simulink model "lab3_simulink"  (R2015a)
settings: Solver=ode45  StartTime=0.0  StopTime=inf  RelTol=1e-3
undefined symbols (not defined in the file or in its folder): currentCFG_lab3_simulink_UB, fdesignblkfcn, gcbh, UB
libraries: dspstat3 x2, gtecHighspeedLib x1, gUSBamplib x1
settings Model: Creator=circuit  LastModifiedBy=circuit

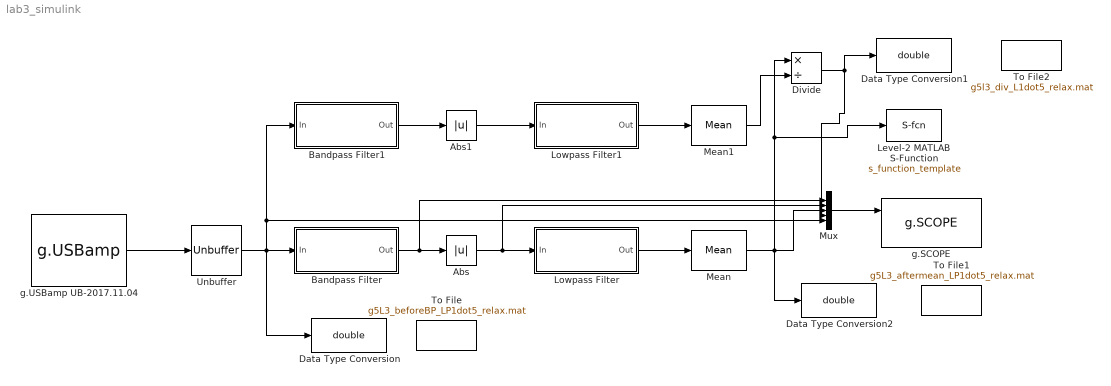
== system lab3_simulink ==
  Abs : Abs
  Abs1 : Abs
  Bandpass Filter : Subsystem  DialogController=fdesignblkfcn  InitFcn=fdesignblkfcn(gcbh, {'InitFcn'});  mask(Bandpass Filter){}
      mask help: Design a bandpass filter
      settings: CopyFcn=fdesignblkfcn(gcbh, {'CopyFcn'});
      mask Help: helpview(mapfilelocation('dsp'), 'dspbandpassfilter');
      mask Display: disp('Bandpass');
  Bandpass Filter1 : Subsystem  DialogController=fdesignblkfcn  InitFcn=fdesignblkfcn(gcbh, {'InitFcn'});  mask(Bandpass Filter){}
      mask help: Design a bandpass filter
      settings: CopyFcn=fdesignblkfcn(gcbh, {'CopyFcn'});
      mask Help: helpview(mapfilelocation('dsp'), 'dspbandpassfilter');
      mask Display: disp('Bandpass');
  Data Type Conversion : DataTypeConversion  OutDataTypeStr=double
  Data Type Conversion1 : DataTypeConversion  OutDataTypeStr=double
  Data Type Conversion2 : DataTypeConversion  OutDataTypeStr=double
  Divide : Product  Inputs=*/
  Level-2 MATLAB S-Function : M-S-Function  FunctionName=s_function_template
  Lowpass Filter : Subsystem  DialogController=fdesignblkfcn  InitFcn=fdesignblkfcn(gcbh, {'InitFcn'});  mask(Lowpass Filter){}
      mask help: Design a lowpass filter
      settings: CopyFcn=fdesignblkfcn(gcbh, {'CopyFcn'});
      mask Help: helpview(mapfilelocation('dsp'), 'dsplowpassfilter');
      mask Display: disp('Lowpass')
  Lowpass Filter1 : Subsystem  DialogController=fdesignblkfcn  InitFcn=fdesignblkfcn(gcbh, {'InitFcn'});  mask(Lowpass Filter){}
      mask help: Design a lowpass filter
      settings: CopyFcn=fdesignblkfcn(gcbh, {'CopyFcn'});
      mask Help: helpview(mapfilelocation('dsp'), 'dsplowpassfilter');
      mask Display: disp('Lowpass')
  Mean : dspstat3/Mean  run=off  reset_popup=None  InputProcessing=Columns as channels (frame based)  directionMode=Each row  dimension=1  treatSBRowAsCol=off  roiEnable=off  roiType=Rectangles  roiPortion=Entire ROI  roiOutput=Individual statistics for each ROI  roiFlag=off  outputDataTypeStr=Inherit: Same as accumulator  outputLastDataTypeStr=Inherit: Same as accumulator  outputMin=[]  outputMax=[]  roundingMode=Floor  overflowMode=off
  Mean1 : dspstat3/Mean  run=off  reset_popup=None  InputProcessing=Columns as channels (frame based)  directionMode=Each row  dimension=1  treatSBRowAsCol=off  roiEnable=off  roiType=Rectangles  roiPortion=Entire ROI  roiOutput=Individual statistics for each ROI  roiFlag=off  outputDataTypeStr=Inherit: Same as accumulator  outputLastDataTypeStr=Inherit: Same as accumulator  outputMin=[]  outputMax=[]  roundingMode=Floor  overflowMode=off
  Mux : Mux  Inputs=5
  To File : ToFile  Filename=g5L3_beforeBP_LP1dot5_relax.mat
  To File1 : ToFile  Filename=g5L3_aftermean_LP1dot5_relax.mat
  To File2 : ToFile  Filename=g5l3_div_L1dot5_relax.mat
  Unbuffer : Unbuffer  SampleBasedProcessing=Same as frame based
  g.SCOPE : gtecHighspeedLib/g.SCOPE
  g.USBamp UB-2017.11.04 : gUSBamplib/g.USBamp  cfg=currentCFG_lab3_simulink_UB-2017.11.04.cfg  snr=UB-2017.11.04
  wires:
  g.USBamp UB-2017.11.04/1 -> Unbuffer/1
  Unbuffer/1 -> Mux/5, Bandpass Filter1/1(In), Data Type Conversion/1, Bandpass Filter/1(In)
  Bandpass Filter/1(Out) -> Mux/1, Abs/1
  Abs/1 -> Mux/2, Lowpass Filter/1(In)
  Lowpass Filter/1(Out) -> Mean/1
  Mean/1 -> Data Type Conversion2/1, Level-2 MATLAB S-Function/1, Divide/1, Mux/3
  Mux/1 -> g.SCOPE/1
  Bandpass Filter1/1(Out) -> Abs1/1
  Abs1/1 -> Lowpass Filter1/1(In)
  Lowpass Filter1/1(Out) -> Mean1/1
  Mean1/1 -> Divide/2
  Divide/1 -> Mux/4, Data Type Conversion1/1

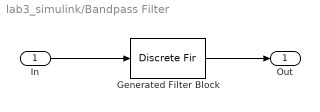
== system lab3_simulink/Bandpass Filter ==
  In : Inport
  Generated Filter Block : DiscreteFir  Tag=BlockMethodSubSystem  Coefficients=[-9.7066588284270048e-20 -1.9044423256952615e-05 -3.5042718823172766e-05 -4.4807719825143353e-05 -4.5567280109715214e-05 -3.5219071376037001e-05 -1.2566832640538831e-05 2.2477748850210183e-05 6.8746329856826839e-05 0.00012373897417179035 0.00018364330584267209 0.00024346501349722092 0.00029728073065491296 0.00033861492674996772 0.00036093040336402629 0.00035820828397517676 0.00032557941097418372 0.0002599565024307643 0.00016060705750857635 2.9602505805759997e-05 -0.00012791919221331879 -0.0003037315778843503 -0.00048677665569194672 -0.00066371693142762433 -0.00081977170567080506 -0.00093979727898122259 -0.001009541477783594 -0.0010169770659436866 -0.0009535992818404458 -0.00081556269315769165 -0.00060453385821604357 -0.0003281500071823974 1.3026996240236752e-18 0.00036091922099598179 0.00073127225101849466 0.0010849327740993554 0.0013949112623725371 0.0016355204203750049 0.0017846012484941276 0.0018256120596552639 0.0017493796388294641 0.001555327713823481 0.0012520329610216285 0.0008570109488230908 0.0003956999203308493 -0.00010031627534579806 -0.00059573006989686742 -0.0010543920094732372 -0.0014424118496333066 -0.0017312017957872362 -0.0019001726269555566 -0.0019388084332589079 -0.0018478882200996666 -0.0016396904076892227 -0.001337104385200843 -0.00097167455182888224 -0.00058070771915937872 -0.00020367438747929246 0.00012178182357201864 0.00036385360046769139 0.0005001989403861936 0.00052080130177256526 0.00042972187623116194 0.00024549074262117919 -6.5519947091882275e-19 -0.0002641002738728534 -0.00049735500687277676 -0.00064851427405487275 -0.00067018306520218889 -0.00052459840768443052 -0.0001889689641773141 0.00034019037963081895 0.0010442453309613309 0.001881563110656567 0.0027888299531657881 0.0036846416750790827 0.0044752368273439759 0.005062031623457793 0.0053504212256518489 0.0052591518963344946 0.0047294598397193298 0.0037331285176027498 0.0022786450626614109 0.00041474033817082845 -0.0017692281561480106 -0.0041463568556569328 -0.006558769024306554 -0.0088274099101692555 -0.010764498450602051 -0.012187803187946064 -0.012935697127694851 -0.012881808406232986 -0.011948036879107893 -0.010114760172307535 -0.0074272073597878765 -0.0039972267037172481 5.2492950851645509e-18 0.0043343631135675798 0.0087340107907784674 0.012902574048254914 0.016539329842932604 0.019360910578682729 0.021122975864728812 0.021640187116165964 0.020802878702137963 0.018589001722594856 0.015070218552972236 0.01041142840998025 0.0048634779709632522 -0.0012506785757137296 -0.0075555979048902606 -0.013647507136755674 -0.019121382890505238 -0.023599056579892485 -0.026756318585830479 -0.02834701119854131 -0.028222271249457628 -0.026343398434246216 -0.02278726318863793 -0.017743697271463996 -0.011504891841311345 -0.0044474179341587091 0.0029919623316966384 0.010345051741279927 0.017143542281197032 0.022950697652655314 0.027391135842824384 0.030176573770733611 0.031125676488437466 0.030176573770733611 0.027391135842824384 0.022950697652655314 0.017143542281197032 0.010345051741279927 0.0029919623316966384 -0.0044474179341587091 -0.011504891841311345 -0.017743697271463996 -0.02278726318863793 -0.026343398434246216 -0.028222271249457628 -0.02834701119854131 -0.026756318585830479 -0.023599056579892485 -0.019121382890505238 -0.013647507136755674 -0.0075555979048902606 -0.0012506785757137296 0.0048634779709632522 0.01041142840998025 0.015070218552972236 0.018589001722594856 0.020802878702137963 0.021640187116165964 0.021122975864728812 0.019360910578682729 0.016539329842932604 0.012902574048254914 0.0087340107907784674 0.0043343631135675798 5.2492950851645509e-18 -0.0039972267037172481 -0.0074272073597878765 -0.010114760172307535 -0.011948036879107893 -0.012881808406232986 -0.012935697127694851 -0.012187803187946064 -0.010764498450602051 -0.0088274099101692555 -0.006558769024306554 -0.0041463568556569328 -0.0017692281561480106 0.00041474033817082845 0.0022786450626614109 0.0037331285176027498 0.0047294598397193298 0.0052591518963344946 ...(+1817 chars)]  InputProcessing=Columns as channels (frame based)
  Out : Outport
  wires:
  In/1 -> Generated Filter Block/1
  Generated Filter Block/1 -> Out/1

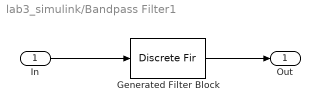
== system lab3_simulink/Bandpass Filter1 ==
  In : Inport
  Generated Filter Block : DiscreteFir  Tag=BlockMethodSubSystem  Coefficients=[-3.9043503106395059e-19 -7.5114923761997586e-05 -0.00012970926989761377 -0.00014606949442778406 -0.00011439896508069259 -3.5260344443637117e-05 8.0051557029435554e-05 0.00021140930249864958 0.000333790689790907 0.00042258113740490207 0.0004592101397287817 0.00043590560812563524 0.00035840430730046821 0.00024577958330473281 0.00012710940297959957 3.5414445181371547e-05 -4.995904333114398e-20 3.8863334376989846e-05 0.00015302162022515448 0.00032437590336606404 0.0005180515405703327 0.00068915525114254914 0.00079277447262141975 0.00079508692530240064 0.00068291437643216318 0.00046913655038040986 0.00019213465104790252 -9.1254063378733906e-05 -0.00031819201546482844 -0.00043512694543481635 -0.00041232096551297316 -0.0002538426644640838 3.5814836249778259e-18 0.00027919151213974422 0.00049876260278053136 0.00057884389263584697 0.00046544668648687939 0.00014675639116760108 -0.00033964304160326449 -0.00091132562644572401 -0.0014573282987569898 -0.0018631749037373697 -0.0020390866299198735 -0.00194452483268953 -0.0016025191355891963 -0.001099237431152839 -0.00056759386496819269 -0.00015763094535208865 0 -0.00017115615086961137 -0.00066918665182910024 -0.0014072608476174431 -0.0022278305628302426 -0.0029357410908228995 -0.0033435027143655905 -0.0033183670710667476 -0.0028195662306453326 -0.0019156126568000984 -0.00077575828959283732 0.00036427999882693573 0.0012557747791148068 0.0016977695616763443 0.0015905989231668213 0.00096826342113219891 -2.6354364596816659e-18 -0.0010416630459124207 -0.0018409403433254869 -0.0021141033846413331 -0.00168252853558822 -0.00052521318214320391 0.0012037448293721349 0.0031995824561332122 0.0050702251314133735 0.0064257287141921728 0.0069736219711172753 0.0065970709591041173 0.0053953855387002675 0.0036742149409364814 0.0018842658898869677 0.00051994874173862549 0 0.00055810037639090549 0.0021710251393396987 0.0045446075659693009 0.007165080986318643 0.0094079239968750117 0.010681746122149461 0.010574625825446118 0.0089674121418749399 0.0060840184071469412 0.0024619054376523448 -0.0011558936775474709 -0.0039867583877307607 -0.0053965252880086474 -0.0050657101633476698 -0.003092081836751504 4.2228921936307396e-18 0.0033528759939696652 0.0059570125198306449 0.0068839068792203315 0.0055187569845934793 0.0017372680468242762 -0.0040200979218537282 -0.010802545357728737 -0.017329928367361164 -0.022268336883116961 -0.024543667872978008 -0.023623130036761086 -0.019696280220295855 -0.013704582830915956 -0.0071987486173472988 -0.0020402937734144686 0 -0.002333132797226467 -0.0094228129569531496 -0.020575338090327674 -0.034025022595054896 -0.047165853317594202 -0.056980799081539031 -0.060596524457473204 -0.055860811648837987 -0.041829167575723386 -0.019058998402915254 0.010357175059788049 0.043039731361273592 0.07481739343065448 0.10138723110404568 0.11902229894830223 0.12519812101626032 0.11902229894830223 0.10138723110404568 0.07481739343065448 0.043039731361273592 0.010357175059788049 -0.019058998402915254 -0.041829167575723386 -0.055860811648837987 -0.060596524457473204 -0.056980799081539031 -0.047165853317594202 -0.034025022595054896 -0.020575338090327674 -0.0094228129569531496 -0.002333132797226467 0 -0.0020402937734144686 -0.0071987486173472988 -0.013704582830915956 -0.019696280220295855 -0.023623130036761086 -0.024543667872978008 -0.022268336883116961 -0.017329928367361164 -0.010802545357728737 -0.0040200979218537282 0.0017372680468242762 0.0055187569845934793 0.0068839068792203315 0.0059570125198306449 0.0033528759939696652 4.2228921936307396e-18 -0.003092081836751504 -0.0050657101633476698 -0.0053965252880086474 -0.0039867583877307607 -0.0011558936775474709 0.0024619054376523448 0.0060840184071469412 0.0089674121418749399 0.010574625825446118 0.010681746122149461 0.0094079239968750117 0.007165080986318643 0.0045446075659693009 0.0021710251393396987 0.00055810037639090549 0 0.00051994874173862549 0.0018842658898869677 0.0036742149409364814 0.0053953855387002675 0.0065970709591041173 ...(+1706 chars)]  InputProcessing=Columns as channels (frame based)
  Out : Outport
  wires:
  In/1 -> Generated Filter Block/1
  Generated Filter Block/1 -> Out/1

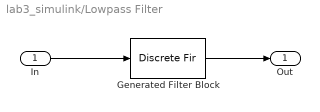
== system lab3_simulink/Lowpass Filter ==
  In : Inport
  Generated Filter Block : DiscreteFir  Tag=BlockMethodSubSystem  Coefficients=[1.4428298688351188e-20 1.45208171766696e-06 2.9191625460814213e-06 4.4049970012497788e-06 5.9133935180921881e-06 7.4482126794738371e-06 9.0133654082074441e-06 1.0612811122812577e-05 1.2250555857839479e-05 1.3930650349583523e-05 1.5657188088038609e-05 1.7434303335956318e-05 1.9266169115897482e-05 2.1156995166181424e-05 2.3111025866657028e-05 2.5132538135237749e-05 2.7225839296160136e-05 2.9395264920942651e-05 3.1645176643039415e-05 3.3979959947197383e-05 3.6404021934544024e-05 3.8921789064445974e-05 4.1537704874194934e-05 4.4256227677590849e-05 4.7081828243506648e-05 5.0018987455532009e-05 5.3072193953806083e-05 5.6245941760161995e-05 5.9544727887716448e-05 6.2973049936051491e-05 6.6535403673141706e-05 7.0236280605195109e-05 7.4080165535581819e-05 7.8071534114035083e-05 8.2214850377317441e-05 8.651456428255206e-05 9.0975109234426682e-05 9.5600899607484595e-05 0.0001003963282647219 0.00010536576407371653 0.00011051354942152003 0.0001158439977295443 0.00012136139096968262 0.00012706997718290485 0.00013297396800156886 0.00013907753617669477 0.00014538481311144461 0.00015189988640205564 0.00015862679738747154 0.00016556953870891733 0.00017273205188065983 0.00018011822487319705 0.00018773188971011259 0.00019557682007983164 0.00020365672896350919 0.00021197526628027701 0.0002205360165510704 0.00022934249658225023 0.00023839815317022907 0.00024770636082830321 0.0002572704195368833 0.00026709355251831266 0.00027717890403744435 0.00028752953722915094 0.00029814843195391652 0.00030903848268266351 0.00032020249641194509 0.00033164319061062744 0.00034336319119917153 0.00035536503056261208 0.00036765114559831707 0.0003802238757995954 0.00039308546137620996 0.00040623804141283194 0.00041968365206646155 0.00043342422480381864 0.00044746158467969812 0.00046179744865725437 0.00047643342397117616 0.00049137100653468154 0.00050661157939125266 0.00052215641121200267 0.00053800665483955796 0.00055416334587930457 0.00057062740133883758 0.00058739961831642709 0.00060448067273929083 0.00062187111815244288 0.00063957138455886719 0.00065758177731173567 0.00067590247605937262 0.00069453353374364314 0.00071347487565241133 0.00073272629852670233 0.00075228746972316328 0.00077215792643240224 0.00079233707495375701 0.0008128241900270159 0.00083361841422158797 0.00085471875738359678 0.00087612409614133886 0.00089783317346952781 0.00091984459831270988 0.00094215684526821456 0.00096476825432897483 0.00098767703068652207 0.0010108812445944334 0.0010343788312924805 0.001058167590991699 0.0010822451889205716 0.0011066091554324852 0.0011312568861745979 0.0011561856423182159 0.0011813925508507587 0.0012068746049293559 0.0012326286642960896 0.0012586514557548691 0.0012849395737099 0.0013114894807656631 0.0013382975083883106 0.0013653598576283397 0.0013926725999043852 0.0014202316778479387 0.0014480329062087722 0.0014760719728208135 0.0015043444396281973 0.0015328457437711754 0.001561571198731555 0.0015905159955372915 0.0016196752040258393 0.001649043774165836 0.0016786165374366667 0.0017083882082654166 0.0017383533855207178 0.0017685065540629331 0.0017988420863501169 0.0018293542440991598 0.0018600371800014915 0.0018908849394926963 0.001921891462575358 0.0019530505856944402 0.0019843560436644627 0.0020158014716477306 0.0020473804071828253 0.0020790862922625583 0.0021109124754605506 0.0021428522141055924 0.0021748986765028917 0.002207044944201317 0.0022392840143057066 0.0022716088018332921 0.0023040121421132637 0.0023364867932284933 0.0023690254384983803 0.0024016206890018067 0.0024342650861391263 0.0024669511042321214 0.0024996711531608206 0.0025324175810360746 0.002565182676906736 0.0025979586735003163 0.0026307377499959206 0.0026635120348282985 0.0026962736085217849 0.0027290145065529321 0.0027617267222405763 0.0027944022096621146 0.0028270328865946928 0.0028596106374800699 0.0028921273164118281 0.0029245747501436526 0.0029569447411173545 0.0029892290705093136 0.0030214195012940033 0.0030535077813232574 0.0030854856464199156 0.0031173448234844878 ...(+7462 chars)]  InputProcessing=Columns as channels (frame based)
  Out : Outport
  wires:
  In/1 -> Generated Filter Block/1
  Generated Filter Block/1 -> Out/1

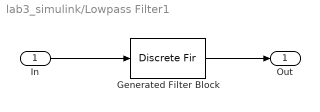
== system lab3_simulink/Lowpass Filter1 ==
  In : Inport
  Generated Filter Block : DiscreteFir  Tag=BlockMethodSubSystem  Coefficients=[1.4428298688351188e-20 1.45208171766696e-06 2.9191625460814213e-06 4.4049970012497788e-06 5.9133935180921881e-06 7.4482126794738371e-06 9.0133654082074441e-06 1.0612811122812577e-05 1.2250555857839479e-05 1.3930650349583523e-05 1.5657188088038609e-05 1.7434303335956318e-05 1.9266169115897482e-05 2.1156995166181424e-05 2.3111025866657028e-05 2.5132538135237749e-05 2.7225839296160136e-05 2.9395264920942651e-05 3.1645176643039415e-05 3.3979959947197383e-05 3.6404021934544024e-05 3.8921789064445974e-05 4.1537704874194934e-05 4.4256227677590849e-05 4.7081828243506648e-05 5.0018987455532009e-05 5.3072193953806083e-05 5.6245941760161995e-05 5.9544727887716448e-05 6.2973049936051491e-05 6.6535403673141706e-05 7.0236280605195109e-05 7.4080165535581819e-05 7.8071534114035083e-05 8.2214850377317441e-05 8.651456428255206e-05 9.0975109234426682e-05 9.5600899607484595e-05 0.0001003963282647219 0.00010536576407371653 0.00011051354942152003 0.0001158439977295443 0.00012136139096968262 0.00012706997718290485 0.00013297396800156886 0.00013907753617669477 0.00014538481311144461 0.00015189988640205564 0.00015862679738747154 0.00016556953870891733 0.00017273205188065983 0.00018011822487319705 0.00018773188971011259 0.00019557682007983164 0.00020365672896350919 0.00021197526628027701 0.0002205360165510704 0.00022934249658225023 0.00023839815317022907 0.00024770636082830321 0.0002572704195368833 0.00026709355251831266 0.00027717890403744435 0.00028752953722915094 0.00029814843195391652 0.00030903848268266351 0.00032020249641194509 0.00033164319061062744 0.00034336319119917153 0.00035536503056261208 0.00036765114559831707 0.0003802238757995954 0.00039308546137620996 0.00040623804141283194 0.00041968365206646155 0.00043342422480381864 0.00044746158467969812 0.00046179744865725437 0.00047643342397117616 0.00049137100653468154 0.00050661157939125266 0.00052215641121200267 0.00053800665483955796 0.00055416334587930457 0.00057062740133883758 0.00058739961831642709 0.00060448067273929083 0.00062187111815244288 0.00063957138455886719 0.00065758177731173567 0.00067590247605937262 0.00069453353374364314 0.00071347487565241133 0.00073272629852670233 0.00075228746972316328 0.00077215792643240224 0.00079233707495375701 0.0008128241900270159 0.00083361841422158797 0.00085471875738359678 0.00087612409614133886 0.00089783317346952781 0.00091984459831270988 0.00094215684526821456 0.00096476825432897483 0.00098767703068652207 0.0010108812445944334 0.0010343788312924805 0.001058167590991699 0.0010822451889205716 0.0011066091554324852 0.0011312568861745979 0.0011561856423182159 0.0011813925508507587 0.0012068746049293559 0.0012326286642960896 0.0012586514557548691 0.0012849395737099 0.0013114894807656631 0.0013382975083883106 0.0013653598576283397 0.0013926725999043852 0.0014202316778479387 0.0014480329062087722 0.0014760719728208135 0.0015043444396281973 0.0015328457437711754 0.001561571198731555 0.0015905159955372915 0.0016196752040258393 0.001649043774165836 0.0016786165374366667 0.0017083882082654166 0.0017383533855207178 0.0017685065540629331 0.0017988420863501169 0.0018293542440991598 0.0018600371800014915 0.0018908849394926963 0.001921891462575358 0.0019530505856944402 0.0019843560436644627 0.0020158014716477306 0.0020473804071828253 0.0020790862922625583 0.0021109124754605506 0.0021428522141055924 0.0021748986765028917 0.002207044944201317 0.0022392840143057066 0.0022716088018332921 0.0023040121421132637 0.0023364867932284933 0.0023690254384983803 0.0024016206890018067 0.0024342650861391263 0.0024669511042321214 0.0024996711531608206 0.0025324175810360746 0.002565182676906736 0.0025979586735003163 0.0026307377499959206 0.0026635120348282985 0.0026962736085217849 0.0027290145065529321 0.0027617267222405763 0.0027944022096621146 0.0028270328865946928 0.0028596106374800699 0.0028921273164118281 0.0029245747501436526 0.0029569447411173545 0.0029892290705093136 0.0030214195012940033 0.0030535077813232574 0.0030854856464199156 0.0031173448234844878 ...(+7462 chars)]  InputProcessing=Columns as channels (frame based)
  Out : Outport
  wires:
  In/1 -> Generated Filter Block/1
  Generated Filter Block/1 -> Out/1
